simulink model "radar"  (R2018a)
settings: Solver=ode4  StartTime=0.0  StopTime=10.0  FixedStep=0.001  RelTol=1e-3
libraries: simulink x1
settings Model: Creator=q  LastModifiedBy=q

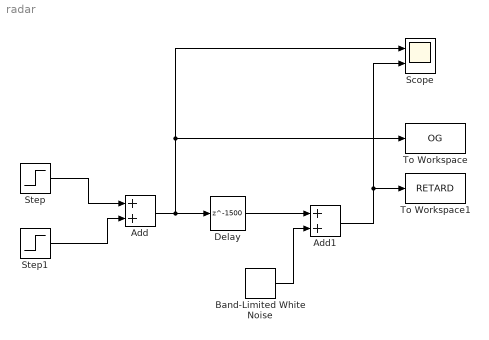
== system radar ==
  Add : Sum
  Add1 : Sum
  Band-Limited White Noise : simulink/Sources/Band-Limited White Noise  Cov=[0.01]  Ts=0.01  seed=[1]
  Delay : Delay  DelayLength=1500
  Scope : Scope  NumInputPorts=2
  Step : Step  After=10  SampleTime=0.001
  Step1 : Step  Time=2  After=-10  SampleTime=0.001
  To Workspace : ToWorkspace  VariableName=OG  SampleTime=-1
  To Workspace1 : ToWorkspace  VariableName=RETARD  SampleTime=-1
  wires:
  Step/1 -> Add/1
  Step1/1 -> Add/2
  Add/1 -> Delay/1, To Workspace/1, Scope/1
  Delay/1 -> Add1/1
  Band-Limited White Noise/1 -> Add1/2
  Add1/1 -> Scope/2, To Workspace1/1
